simulink subsystem "VehicleBody6DOFSSC"  (R2023b)
settings: Solver=VariableStepAuto  StartTime=0.0  StopTime=10.0  RelTol=1e-3
undefined symbols (not defined in the file): EnvAirDen, PlntVehAeroDragCff, PlntVehAeroFrntArea, PlntVehAeroLiftCff, PlntVehCGHgtAxl, PlntVehDstCGFrntAxl, PlntVehDstCGRearAxl, PlntVehInitLatPos, PlntVehInitVertPos, PlntVehMass, PlntVehMultiBody, PlntVehPitchMomentInertia, PlntVehRollMomentInertia, PlntVehYawMomentInertia, X, Y, Z
libraries: nesl_utility x44, sm_lib x42, sharedtransform x12, fl_lib x4, vehdynlibeomcommon x3, matrix_library x1
(part 3 of 3)

== system VehicleBody6DOFSSC/Body Sensor/InertFrm/Geom/vehBus_Values_InertFrm_Geom_Ang ==
  Signal Specification1 : SignalSpecification  Unit=rad
  Signal Specification2 : SignalSpecification  Unit=rad
  Signal Specification4 : SignalSpecification  Unit=rad
  busOut : BusCreator  Inputs=3
  phi : Constant  Value=zeros([1,1])  SampleTime=-1
  psi : Constant  Value=zeros([1,1])  SampleTime=-1
  theta : Constant  Value=zeros([1,1])  SampleTime=-1
  Out1 : Outport
  wires:
  theta/1 -> Signal Specification1/1  "theta"
  psi/1 -> Signal Specification2/1  "psi"
  phi/1 -> Signal Specification4/1  "phi"
  busOut/1 -> Out1/1
  Signal Specification4/1 -> busOut/1  "phi"
  Signal Specification1/1 -> busOut/2  "theta"
  Signal Specification2/1 -> busOut/3  "psi"

== system VehicleBody6DOFSSC/Body Sensor/InertFrm/Geom/vehBus_Values_InertFrm_Geom_Disp ==
  In : Inport
  Bus Selector : BusSelector  OutputSignals=X,Y,Z
  busOut : BusCreator  Inputs=3
  Out1 : Outport
  wires:
  busOut/1 -> Out1/1
  Bus Selector/1 -> busOut/1  "<X>"
  Bus Selector/3 -> busOut/3  "<Z>"
  In/1 -> Bus Selector/1
  Bus Selector/2 -> busOut/2  "<Y>"

== system VehicleBody6DOFSSC/Body Sensor/InertFrm/Geom/vehBus_Values_InertFrm_Geom_Vel ==
  In : Inport
  Bus Selector : BusSelector  OutputSignals=Xdot,Ydot,Zdot
  busOut : BusCreator  Inputs=3
  Out1 : Outport
  wires:
  busOut/1 -> Out1/1
  Bus Selector/3 -> busOut/3  "<Zdot>"
  Bus Selector/2 -> busOut/2  "<Ydot>"
  Bus Selector/1 -> busOut/1  "<Xdot>"
  In/1 -> Bus Selector/1

== system VehicleBody6DOFSSC/Body Sensor/InertFrm/Hitch/vehBus_Values_InertFrm_Hitch_Disp ==
  Signal Specification1 : SignalSpecification  Unit=m
  Signal Specification2 : SignalSpecification  Unit=m
  Signal Specification4 : SignalSpecification  Unit=m
  X : Constant  Value=zeros([1,1])  SampleTime=-1
  Y : Constant  Value=zeros([1,1])  SampleTime=-1
  Z : Constant  Value=zeros([1,1])  SampleTime=-1
  busOut : BusCreator  Inputs=3
  Out1 : Outport
  wires:
  busOut/1 -> Out1/1
  Y/1 -> Signal Specification1/1  "Y"
  X/1 -> Signal Specification4/1  "X"
  Z/1 -> Signal Specification2/1  "Z"
  Signal Specification4/1 -> busOut/1  "X"
  Signal Specification1/1 -> busOut/2  "Y"
  Signal Specification2/1 -> busOut/3  "Z"

== system VehicleBody6DOFSSC/Body Sensor/InertFrm/Hitch/vehBus_Values_InertFrm_Hitch_Vel ==
  Signal Specification1 : SignalSpecification  Unit=m/s
  Signal Specification2 : SignalSpecification  Unit=m/s
  Signal Specification4 : SignalSpecification  Unit=m/s
  Xdot : Constant  Value=zeros([1,1])  SampleTime=-1
  Ydot : Constant  Value=zeros([1,1])  SampleTime=-1
  Zdot : Constant  Value=zeros([1,1])  SampleTime=-1
  busOut : BusCreator  Inputs=3
  Out1 : Outport
  wires:
  Zdot/1 -> Signal Specification2/1  "Zdot"
  busOut/1 -> Out1/1
  Ydot/1 -> Signal Specification1/1  "Ydot"
  Xdot/1 -> Signal Specification4/1  "Xdot"
  Signal Specification4/1 -> busOut/1  "Xdot"
  Signal Specification1/1 -> busOut/2  "Ydot"
  Signal Specification2/1 -> busOut/3  "Zdot"

== system VehicleBody6DOFSSC/Body Sensor/InertFrm/RearAxl/vehBus_Values_InertFrm_RearAxl_Disp ==
  In : Inport
  Bus Selector : BusSelector  OutputSignals=X,Y,Z
  busOut : BusCreator  Inputs=3
  Out1 : Outport
  wires:
  busOut/1 -> Out1/1
  In/1 -> Bus Selector/1
  Bus Selector/3 -> busOut/3  "<Z>"
  Bus Selector/2 -> busOut/2  "<Y>"
  Bus Selector/1 -> busOut/1  "<X>"

== system VehicleBody6DOFSSC/Body Sensor/InertFrm/RearAxl/vehBus_Values_InertFrm_RearAxl_Vel ==
  In : Inport
  Bus Selector : BusSelector  OutputSignals=Xdot,Ydot,Zdot
  busOut : BusCreator  Inputs=3
  Out1 : Outport
  wires:
  busOut/1 -> Out1/1
  Bus Selector/1 -> busOut/1  "<Xdot>"
  Bus Selector/2 -> busOut/2  "<Ydot>"
  In/1 -> Bus Selector/1
  Bus Selector/3 -> busOut/3  "<Zdot>"
